simulink subsystem "FluxMapID_6ph"  (R2022b)
settings: Solver=VariableStepAuto  StartTime=0.0  StopTime=10.0  RelTol=1e-3
libraries: Subchart_FluxMapID_references x3
settings Model: Creator=valen  LastModifiedBy=valen
settings DebuggingCC: UnconnectedInputMsg=warning  UnconnectedOutputMsg=warning  UnconnectedLineMsg=warning
settings ModelReferenceCC: EnableRefExpFcnMdlSchedulingChecks=on
settings RTWCC: DLArmComputeVersion=19.05

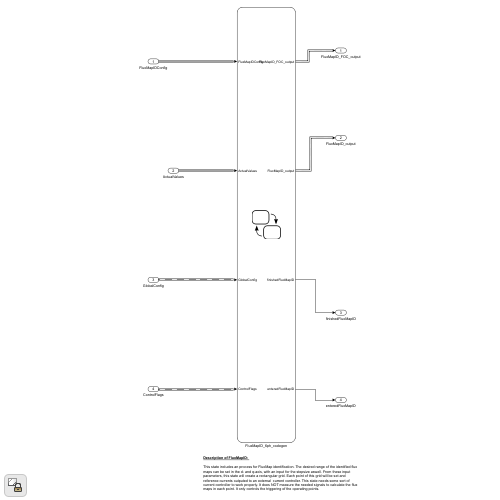
[thumbnail: Simulink's stored preview of the top-level diagram]
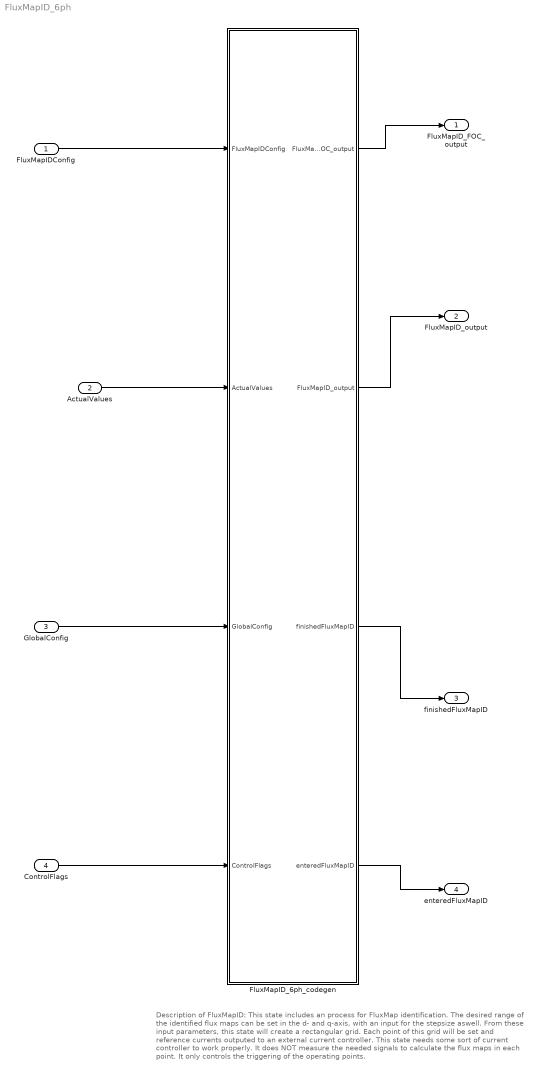
== system FluxMapID_6ph ==
  note: Description of FluxMapID:
      |
      | This state includes an process for FluxMap identification. The desired range of the identified flux maps can be set in the d- and q-axis, with an input for the stepsize aswell. From these input parameters, this state will create a rectangular grid. Each point of this grid will be set and reference currents outputed to an external current controller. This state needs some sort of current controller to work properly. It does NOT measure the needed signals to calculate the flux maps in each point. It only controls the triggering of the operating points.
  FluxMapIDConfig : Inport
  ActualValues : Inport  Port=2
  GlobalConfig : Inport  Port=3
  ControlFlags : Inport  Port=4
  FluxMapID_6ph_codegen : Stateflow chart  TreatAsAtomicUnit=on
      settings: PortSchema="{\"entries\":[{\"content\":{\"sides\":[{\"content\":{\"connectorIds\":[\"In1\",\"In2\",\"In3\",\"In4\"]},\"type\":\"ConnectorPlacement.EquallySpacedRectSide\",\"uuid\":\"981d5bbf-03cd-4404-8840-685ce2b7a497\"},{\"content\":{\"connectorIds\":[\"Out3\",\"Out4\",\"Out1\",\"Out2\"],\"side\":\"RIGHT\"},\"type\":\"ConnectorPlacement.EquallySpacedRectSide\",\"uuid\":\"92ae37cc-cac4-4d7b-af20-0fade983881b\"},{\"content\":{\"connectorIds\":[],\"side\":\"TOP\"},\"type\":\"ConnectorPlacement.EquallySpacedRectSide\",\"uuid\":\"d233b8d0-893b-4073-8e4e-3204ab89fedb\"}]},\"type\":\"ConnectorPlacement.EquallySpacedConnector\",\"uuid\":\"28ed47dd-3acf-49aa-8a06-7eb7a90c4cf1\"}],\"packageUris\":[\"http://schema.mathworks.com/mf0/Connector/R2020b\"],\"version\":\"1.0\"}"
  FluxMapID_FOC_output : Outport
  FluxMapID_output : Outport  Port=2
  finishedFluxMapID : Outport  Port=3
  enteredFluxMapID : Outport  Port=4
  wires:
  ActualValues/1 -> FluxMapID_6ph_codegen/2(ActualValues)
  FluxMapID_6ph_codegen/2(enteredFluxMapID) -> enteredFluxMapID/1
  FluxMapIDConfig/1 -> FluxMapID_6ph_codegen/1(FluxMapIDConfig)
  FluxMapID_6ph_codegen/4(FluxMapID_output) -> FluxMapID_output/1
  FluxMapID_6ph_codegen/3(FluxMapID_FOC_output) -> FluxMapID_FOC_output/1
  GlobalConfig/1 -> FluxMapID_6ph_codegen/3(GlobalConfig)
  FluxMapID_6ph_codegen/1(finishedFluxMapID) -> finishedFluxMapID/1
  ControlFlags/1 -> FluxMapID_6ph_codegen/4(ControlFlags)

== stateflow chart FluxMapID_6ph/FluxMapID_6ph_codegen ==
  settings: updateMethod=DISCRETE  sampleTime=1/d_f_states
  note: Flux Map identification
  state AMMstate
    entry:
    finishedFluxMapID=false;
    enteredFluxMapID = true;
    fun_R_s_array(:)=FluxMapIDConfig.R_s_ref;
    during:
    FluxMapID_output.WindingTemp = ActualValues.average_winding_temp;
    if(FluxMapIDConfig.start_FM_ID==1)
    if(FluxMapIDConfig.identR == 1)
    if(FluxMapID_FOC_output.activeState ~= 403)
    FluxMapID_output.R_s = identRes;
    else
    fun_i_R_online = single(0);
    end
    if(FluxMapIDConfig.R_s_ref ~= 0.0 && FluxMapIDConfig.Temp_ref ~= 0.0)
    FluxMapID_output.WindingTemp = ((FluxMapID_output.R_s/FluxMapIDConfig.R_s_ref)-1)....
    *254.453+FluxMapIDConfig.Temp_ref;
    end
    end
    if(FluxMapIDConfig.identR == 0)
    fun_i_R_online = single(0.0);
    FluxMapID_output.WindingTemp= FluxMapIDConfig.lower_meas_temp;
    end
    else
    FluxMapID_output.R_s = FluxMapIDConfig.R_s_ref*...
    (single(1)+TEMP_COEFFICIENT*(FluxMapID_output.WindingTemp - FluxMapIDConfig.Temp_ref));
    fun_i_R_online = single(0);
    end
    exit:
    counter = uint32(1);
    finishedFluxMapID=boolean(1);
    enteredFluxMapID = boolean(0);
    state Wait_select_subsystem
      entry:
      FluxMapID_FOC_output.activeState = uint16(400);
      FluxMapID_FOC_output.resetIntegrator = true;
      i_q_ref_AMM = single(0);
      i_d_ref_AMM = single(0);
      repetition_counter = uint32(0);
      reset_FOC_out;
      reset_logging_out;
      exit:
      switch (FluxMapIDConfig.selected_subsystem)
      case 1
      FluxMapID_FOC_output.PI_subsystem = 0x0003;
      FluxMapID_FOC_output.resonant_subsystem = 0x0001;
      FluxMapID_FOC_output.setpoint_filter = 0x0001;
      case 2
      FluxMapID_FOC_output.PI_subsystem = 0x0003;
      FluxMapID_FOC_output.resonant_subsystem = 0x0002;
      FluxMapID_FOC_output.setpoint_filter = 0x0002
      case 3
      FluxMapID_FOC_output.PI_subsystem = 0x0004;
      FluxMapID_FOC_output.resonant_subsystem = 0x0004;
      FluxMapID_FOC_output.setpoint_filter = 0x0004;
      otherwise
      FluxMapID_FOC_output.PI_subsystem = 0x0000;
      FluxMapID_FOC_output.resonant_subsystem = 0x0000;
      end
    state IdentificationDQ
      entry:
      FluxMapID_output.psi_array = [0;0;0;0];
      FluxMapID_FOC_output.resetIntegrator = false;
      FluxMapID_FOC_output.enableFOC_current = true;
      during:
      if(FluxMapIDConfig.start_FM_ID==true)
      FluxMapID_FOC_output.i_dq_ref.d=i_d_ref_AMM;
      FluxMapID_FOC_output.i_dq_ref.q=i_q_ref_AMM;
      FluxMapID_FOC_output.i_xy_ref.d = fun_i_R_online;
      fun_actual_v=ActualValues.v_xy_rotating.d;
      fun_actual_i=ActualValues.i_xy_rotating.d;
      else
      FluxMapID_FOC_output.i_dq_ref.d = single(0);
      FluxMapID_FOC_output.i_dq_ref.q = single(0);
      FluxMapID_FOC_output.i_xy_ref.d = single(0);
      end
      if(finished_calculation)
      FluxMapID_output.psi_array(1)=mean_currents.d;
      FluxMapID_output.psi_array(2)=mean_currents.q;
      FluxMapID_output.psi_array(3)=flux(mean_voltages.q, mean_currents.q,...
      mean_omega_el, FluxMapID_output.R_s);
      FluxMapID_output.psi_array(4)=single(-1)*flux(mean_voltages.d, mean_currents.d,...
      mean_omega_el, FluxMapID_output.R_s);
      FluxMapID_output.array_index = repetition_counter;
      end
      state Fluxmap
      state waitState
        entry:
        FluxMapID_FOC_output.activeState = uint16(405);
      730 -> AMMstate.IdentificationDQ.Fluxmap
      705 -> AMMstate.IdentificationDQ.waitState
    state IdentificationXY
      entry:
      FluxMapID_output.psi_array = [0;0;0;0];
      FluxMapID_FOC_output.resetIntegrator = false;
      FluxMapID_FOC_output.enableFOC_current = true;
      during:
      if(FluxMapIDConfig.start_FM_ID==true)
      FluxMapID_FOC_output.i_xy_ref.d=i_d_ref_AMM+fun_i_R_online;
      FluxMapID_FOC_output.i_xy_ref.q=i_q_ref_AMM;
      fun_actual_v=ActualValues.v_xy_rotating.d;
      fun_actual_i=ActualValues.i_xy_rotating.d;
      else
      FluxMapID_FOC_output.i_xy_ref.d = single(0);
      FluxMapID_FOC_output.i_xy_ref.q = single(0);
      end
      if(finished_calculation)
      FluxMapID_output.psi_array(1)=mean_currents.d;
      FluxMapID_output.psi_array(2)=mean_currents.q;
      FluxMapID_output.psi_array(3)=single(-1)*flux(mean_voltages.q, mean_currents.q, ...
      mean_omega_el, FluxMapID_output.R_s);
      FluxMapID_output.psi_array(4)=flux(mean_voltages.d, mean_currents.d, ...
      mean_omega_el, FluxMapID_output.R_s);
      FluxMapID_output.array_index = repetition_counter;
      end
      state Fluxmap
      state waitState
        entry:
        FluxMapID_FOC_output.activeState = uint16(405);
      739 -> AMMstate.IdentificationXY.Fluxmap
      740 -> AMMstate.IdentificationXY.waitState
    state IdentificationZero
      entry:
      FluxMapID_output.psi_array = [0;0;0;0];
      FluxMapID_FOC_output.resetIntegrator = false;
      FluxMapID_FOC_output.enableFOC_current = true;
      during:
      if(FluxMapIDConfig.start_FM_ID==true)
      FluxMapID_FOC_output.i_zero_ref.d=i_d_ref_AMM+fun_i_R_online;
      FluxMapID_FOC_output.i_zero_ref.q=i_q_ref_AMM;
      fun_actual_v=ActualValues.v_zero_rotating.d;
      fun_actual_i=ActualValues.i_zero_rotating.d;
      else
      FluxMapID_FOC_output.i_zero_ref.d = single(0);
      FluxMapID_FOC_output.i_zero_ref.q = single(0);
      end
      if(finished_calculation)
      FluxMapID_output.psi_array(1)=mean_currents.d;
      FluxMapID_output.psi_array(2)=mean_currents.q;
      FluxMapID_output.psi_array(3)=flux(mean_voltages.q, mean_currents.q, ...
      mean_omega_el, FluxMapID_output.R_s)/single(3);
      FluxMapID_output.psi_array(4)=single(-1)*flux(mean_voltages.d, mean_currents.d, ...
      mean_omega_el, FluxMapID_output.R_s)/single(3);
      FluxMapID_output.array_index = repetition_counter;
      end
      state Fluxmap
      state waitState
        entry:
        FluxMapID_FOC_output.activeState = uint16(405);
      833 -> AMMstate.IdentificationZero.Fluxmap
      818 -> AMMstate.IdentificationZero.waitState
    (default) -> Wait_select_subsystem
    Wait_select_subsystem -> 731 [order 2] : [FluxMapIDConfig.selected_subsystem == 1 && GlobalConfig.ACCEPT==1]
    IdentificationDQ -> Wait_select_subsystem : [FluxMapIDConfig.start_FM_ID==0 && FluxMapIDConfig.selected_subsystem == 0]
    Wait_select_subsystem -> 735 [order 1] : [FluxMapIDConfig.selected_subsystem == 2 && GlobalConfig.ACCEPT==1]
    IdentificationXY -> Wait_select_subsystem : [FluxMapIDConfig.start_FM_ID==0 && FluxMapIDConfig.selected_subsystem == 0]
    Wait_select_subsystem -> 834 [order 3] : [FluxMapIDConfig.selected_subsystem == 3 && GlobalConfig.ACCEPT==1]
    IdentificationZero -> Wait_select_subsystem : [FluxMapIDConfig.start_FM_ID==0 && FluxMapIDConfig.selected_subsystem == 0]
  state Waiting
    entry:
    %wait for activation of
    %FluxMapID
    init;
  note: ---
  Waiting -> AMMstate [order 1] : [ControlFlags.startFluxMapID==1 && ....
      | GlobalConfig.Reset==0 && GlobalConfig.ACCEPT==1]
  (default) -> Waiting
  Waiting -> Waiting [order 2] : [GlobalConfig.Reset==1]{finishedFluxMapID=boolean(0);
      | enteredFluxMapID=boolean(0);}
  AMMstate -> Waiting : [GlobalConfig.Reset==1 || GlobalConfig.FluxMapID==0....
      | || GlobalConfig.enableParameterID==0]
      | {enteredFluxMapID=boolean(0);}
  data: fun function_output; activeState function_output; three_sec_transition_counter function_input; PI_d_ref function_output; PI_q_ref function_output; mean_voltages function_output; mean_omega_el function_output; actual_voltages function_input; omega_el function_input; actual_currents function_input; mean_currents function_output; repetitionCounter function_output; finished_calculation function_output; activeState function_output; three_sec_transition_counter function_input; PI_d_ref function_output; PI_q_ref function_output; mean_voltages function_output; mean_omega_el function_output; actual_voltages function_input; omega_el function_input; actual_currents function_input; mean_currents function_output; repetitionCounter function_output; finished_calculation function_output; activeState function_output; three_sec_transition_counter function_input; PI_d_ref function_output; PI_q_ref function_output; mean_voltages function_output; mean_omega_el function_output; actual_voltages function_input; omega_el function_input; actual_currents function_input; mean_currents function_output; repetitionCounter function_output; finished_calculation function_output; u function_input; i function_input; omega_el function_input; Rs function_input; psi function_output; TEMP_COEFFICIENT constant single size=1 =0.00393; fun_i_R_online local single size=1 =single(0); fun_counter local uint32 size=1 =uint32(0); fun_v1_counter local single size=1 =single(0); fun_v2_counter local single size=1 =single(0); fun_i2_counter local single size=1 =single(0); fun_i1_counter local single size=1 =single(0); fun_R_s_array local single size=20; fun_actual_v local single size=1 =single(0); fun_actual_i local single size=1 =single(0); FluxMapIDConfig input Bus: uz_ParaID_FluxMapIDConfig_t size=1; counter local size=1; finishedFluxMapID output boolean size=1 =false;; enteredFluxMapID output boolean size=1; FluxMapID_FOC_output output Bus: uz_ParaID_Controller_Parameters_output_t size=1; ActualValues input Bus: uz_ParaID_ActualValues_t size=1; GlobalConfig input Bus: uz_ParaID_GlobalConfig_t size=1; ControlFlags input Bus: uz_ParaID_ControlFlags_t size=1; FluxMapID_output output Bus: uz_ParaID_FluxMapID_output_t size=1; three_sec_transition_counter local uint32 size=1; one_sec_transition_counter local uint32 size=1; mean_omega_el local single size=1 =single(0); mean_voltages local Bus: uz_3ph_dq_t size=1; finished_calculation local boolean size=1 =false; i_q_ref_AMM local single size=1; i_d_ref_AMM local single size=1; mean_currents local Bus: uz_3ph_dq_t size=1; repetition_counter local uint32 size=1 =uint32(0)
  function fun = identRes:
    | function fun = identRes 
    | 
    | 	if(fun_counter <= uint32(0.5/GlobalConfig.sampleTimeISR))%meas
    |         fun_i_R_online = single(-FluxMapIDConfig.identRAmp);
    |             if(fun_counter >= uint32(0.4/GlobalConfig.sampleTimeISR) && fun_counter < uint32(0.5/GlobalConfig.sampleTimeISR))
    |                 fun_v1_counter = fun_v1_counter + fun_actual_v;
    |                 fun_i1_counter = fun_i1_counter + fun_actual_i;
    |             end
    | 	end
    |         
    | 	if(fun_counter > uint32(0.5/GlobalConfig.sampleTimeISR) && fun_counter <= uint32(1.0/GlobalConfig.sampleTimeISR))
    |         fun_i_R_online = single(FluxMapIDConfig.identRAmp);
    |             if(fun_counter >= uint32(0.9/GlobalConfig.sampleTimeISR) && fun_counter < uint32(1.0/GlobalConfig.sampleTimeISR))
    |                 fun_v2_counter = fun_v2_counter + fun_actual_v;
    |                 fun_i2_counter = fun_i2_counter + fun_actual_i;
    |             end
    | 	end
    |         
    | 	if(fun_counter == uint32(1.0/GlobalConfig.sampleTimeISR + 1) )
    |         fun_i_R_online = single(-FluxMapIDConfig.identRAmp);
    |         fun_v1_counter=fun_v1_counter/(0.1/GlobalConfig.sampleTimeISR);
    |         fun_i1_counter=fun_i1_counter/(0.1/GlobalConfig.sampleTimeISR);
    |         fun_v2_counter=fun_v2_counter/(0.1/GlobalConfig.sampleTimeISR);
    |         fun_i2_counter=fun_i2_counter/(0.1/GlobalConfig.sampleTimeISR);
    |         fun_R_s_array(1,1) = single((fun_v2_counter-fun_v1_counter)/(fun_i2_counter-fun_i1_counter));
    |         RefreshDataRegister;
    |         FluxMapID_output.R_s = mean(fun_R_s_array);
    |         fun_counter = uint32(1);
    |         fun_v1_counter = single(0);
    |         fun_v2_counter = single(0);
    |         fun_i1_counter = single(0);
    |         fun_i2_counter = single(0);
    | 	end
    |         
    | fun_counter = fun_counter + 1;
    | fun = single(FluxMapID_output.R_s);
    | end
  function psi = flux(u, i, omega_el, Rs):
    | function psi = flux(u, i, omega_el, Rs) 
    | psi = (u-Rs*i)/omega_el;
    | end
  function RefreshDataRegister:
    | function RefreshDataRegister
    | 
    | m=length(fun_R_s_array);
    |     for k= uint16(0):uint16(m-2)
    |         fun_R_s_array(m-k)=fun_R_s_array(m-(k+1));
    |     end
    | 
    | end
  function reset_FOC_out:
    | function reset_FOC_out
    | FluxMapID_FOC_output.setpoint_filter = 0x0000;
    | FluxMapID_FOC_output.i_dq_ref.d = single(0);
    | FluxMapID_FOC_output.i_dq_ref.q = single(0);
    | FluxMapID_FOC_output.i_xy_ref.d = single(0);
    | FluxMapID_FOC_output.i_xy_ref.q = single(0);
    | FluxMapID_FOC_output.i_zero_ref.d = single(0);
    | FluxMapID_FOC_output.i_zero_ref.q = single(0);
    | FluxMapID_FOC_output.PI_subsystem = 0x0000;
    | FluxMapID_FOC_output.resonant_subsystem = 0x0000;
    | FluxMapID_FOC_output.enableFOC_current = false;
    | end
  function init:
    | function init
    | FluxMapID_FOC_output.enableFOC_current=boolean(0);
    | FluxMapID_output.psi_array = single([0;0;0;0]);
    | one_sec_transition_counter = uint32(1/GlobalConfig.sampleTimeISR);
    | three_sec_transition_counter = uint32(3/GlobalConfig.sampleTimeISR);
    | reset_FOC_out;
    | reset_logging_out;
    | FluxMapID_FOC_output.activeState = uint16(0);
  function reset_logging_out:
    | function reset_logging_out
    | FluxMapID_output.psi_array(1)=single(0);
    | FluxMapID_output.psi_array(2)=single(0);
    | FluxMapID_output.psi_array(3)=single(0);
    | FluxMapID_output.psi_array(4)=single(0);
    | FluxMapID_output.array_index =uint32(0);
